simulink model "nn_12B_with_contracts"  (R2019b)
settings: Solver=FixedStepDiscrete  StartTime=0  StopTime=100  FixedStep=1  RelTol=1e-3  EnableMultiTasking=on
model workspace (MAT data in the model file):
  ContractValidatorBlocksMap = containers.Map
  ContractValidatorBlocksMap.serialization.keys = {'nn_12B_with_contracts/nn_12B_NNSpec/validator'}
  ContractValidatorBlocksMap.serialization.values{1}.block = 'nn_12B_with_contracts/nn_12B_NNSpec/validator'
  ContractValidatorBlocksMap.serialization.values{1}.assumePorts = 0
  ContractValidatorBlocksMap.serialization.values{1}.guaranteePorts = 5
  ContractValidatorBlocksMap.serialization.values{1}.modeBlocksPorts = 0
  ContractValidatorBlocksMap.serialization.values{1}.portHandles.Inport = [1930.00012207 1931.00012207 1932.00012207 1933.00012207 1934.00012207]
  ContractValidatorBlocksMap.serialization.values{1}.portHandles.Outport = 1935.00012207
  ContractValidatorBlocksMap.serialization.values{1}.portHandles.Enable = []
  ContractValidatorBlocksMap.serialization.values{1}.portHandles.Trigger = []
  ContractValidatorBlocksMap.serialization.values{1}.portHandles.State = []
  ContractValidatorBlocksMap.serialization.values{1}.portHandles.LConn = []
  ContractValidatorBlocksMap.serialization.values{1}.portHandles.RConn = []
  ContractValidatorBlocksMap.serialization.values{1}.portHandles.Ifaction = []
  ContractValidatorBlocksMap.serialization.values{1}.portHandles.Reset = []
  ContractValidatorBlocksMap.serialization.values{1}.portConnectivity(1).Type = '1'
  ContractValidatorBlocksMap.serialization.values{1}.portConnectivity(1).Position = [2170 860]
  ContractValidatorBlocksMap.serialization.values{1}.portConnectivity(1).SrcBlock = 233.00012207
  ContractValidatorBlocksMap.serialization.values{1}.portConnectivity(1).SrcPort = 0
  ContractValidatorBlocksMap.serialization.values{1}.portConnectivity(1).DstBlock = []
  ContractValidatorBlocksMap.serialization.values{1}.portConnectivity(1).DstPort = []
  ContractValidatorBlocksMap.serialization.values{1}.portConnectivity(2).Type = '2'
  ContractValidatorBlocksMap.serialization.values{1}.portConnectivity(2).Position = [2170 905]
  ContractValidatorBlocksMap.serialization.values{1}.portConnectivity(2).SrcBlock = 237.00012207
  ContractValidatorBlocksMap.serialization.values{1}.portConnectivity(2).SrcPort = 0
  ContractValidatorBlocksMap.serialization.values{1}.portConnectivity(2).DstBlock = []
  ContractValidatorBlocksMap.serialization.values{1}.portConnectivity(2).DstPort = []
  ContractValidatorBlocksMap.serialization.values{1}.portConnectivity(3).Type = '3'
  ContractValidatorBlocksMap.serialization.values{1}.portConnectivity(3).Position = [2170 950]
  ContractValidatorBlocksMap.serialization.values{1}.portConnectivity(3).SrcBlock = 241.00012207
  ContractValidatorBlocksMap.serialization.values{1}.portConnectivity(3).SrcPort = 0
  ContractValidatorBlocksMap.serialization.values{1}.portConnectivity(3).DstBlock = []
  ContractValidatorBlocksMap.serialization.values{1}.portConnectivity(3).DstPort = []
  ContractValidatorBlocksMap.serialization.values{1}.portConnectivity(4).Type = '4'
  ContractValidatorBlocksMap.serialization.values{1}.portConnectivity(4).Position = [2170 995]
  ContractValidatorBlocksMap.serialization.values{1}.portConnectivity(4).SrcBlock = 245.00012207
  ContractValidatorBlocksMap.serialization.values{1}.portConnectivity(4).SrcPort = 0
  ContractValidatorBlocksMap.serialization.values{1}.portConnectivity(4).DstBlock = []
  ContractValidatorBlocksMap.serialization.values{1}.portConnectivity(4).DstPort = []
  ContractValidatorBlocksMap.serialization.values{1}.portConnectivity(5).Type = '5'
  ContractValidatorBlocksMap.serialization.values{1}.portConnectivity(5).Position = [2170 1040]
  ContractValidatorBlocksMap.serialization.values{1}.portConnectivity(5).SrcBlock = 249.00012207
  ContractValidatorBlocksMap.serialization.values{1}.portConnectivity(5).SrcPort = 0
  ContractValidatorBlocksMap.serialization.values{1}.portConnectivity(5).DstBlock = []
  ContractValidatorBlocksMap.serialization.values{1}.portConnectivity(5).DstPort = []
  ContractValidatorBlocksMap.serialization.values{1}.portConnectivity(6).Type = '1'
  ContractValidatorBlocksMap.serialization.values{1}.portConnectivity(6).Position = [2210 950]
  ContractValidatorBlocksMap.serialization.values{1}.portConnectivity(6).SrcBlock = []
  ContractValidatorBlocksMap.serialization.values{1}.portConnectivity(6).SrcPort = []
  ContractValidatorBlocksMap.serialization.values{1}.portConnectivity(6).DstBlock = 291.00012207
  ContractValidatorBlocksMap.serialization.values{1}.portConnectivity(6).DstPort = 0
  ContractValidatorBlocksMap.serialization.uniformity = 0
  ContractValidatorBlocksMap.serialization.keyType = 'char'
  ContractValidatorBlocksMap.serialization.valueType = 'any'
undefined symbols (not defined in the file): b1, b2, b3, contractAfterSimulation, contractBeforeSimulation, ContractBlock, ContractGuaranteeBlock, ContractValidatorBlock, meaninp, meanout, oostdinp, saveValidatorParameters, stdevout, w1, w2, w3, xinmax, xinmin
libraries: cocosimLibs x4
(part 1 of 2)
settings Model: Creator=niestma  LastModifiedBy=hbourbou
settings DataIOCC: LimitDataPoints=on  SaveFormat=Array  ReturnWorkspaceOutputs=off
settings OptimizationCC: ExpressionDepthLimit=2147483647  LifeSpan=1  EfficientTunableParamExpr=on
settings DebuggingCC: UnderspecifiedInitializationDetection=Classic  MergeDetectMultiDrivingBlocksExec=none  StateNameClashWarn=warning  SFUnexpectedBacktrackingDiag=warning  SFNoUnconditionalDefaultTransitionDiag=warning  SFExecutionAtInitializationDiag=none  ArithmeticOperatorsInVariantConditions=warning
settings HardwareCC: ProdBitPerPointer=32  ProdBitPerSizeT=32  ProdBitPerPtrDiffT=32  ProdLargestAtomicFloat=None  ProdIntDivRoundTo=Undefined  ProdEndianess=Unspecified  ProdWordSize=32  ProdHWDeviceType=32-bit Generic
settings ModelReferenceCC: PropagateSignalLabelsOutOfModel=off
settings SFSimCC: SimUseLocalCustomCode=off  MATLABDynamicMemAlloc=off  CustomCodeUndefinedFunction=UseInterfaceOnly
settings RTWCC: SystemTargetFile=ert.tlc  TemplateMakefile=ert_default_tmf  GenerateReport=on  RTWUseLocalCustomCode=off  IncludeHyperlinkInReport=on  LaunchReport=on
settings CodeAppCC: IgnoreCustomStorageClasses=off  CustomSymbolStrType=$N$R$M  StateflowObjectComments=on  InternalIdentifier=Classic
settings ERTTargetCC: MultiwordLength=2048  GenerateSampleERTMain=on  ERTCustomFileTemplate=example_file_process.tlc  ConvertIfToSwitch=off  SuppressUnreachableDefaultCases=off
settings ConfigComp: CovMetricSettings=dw  CovHtmlReporting=on  CovSaveCumulativeToWorkspaceVar=on  CovSaveSingleToWorkspaceVar=on  CovExternalEMLEnable=off

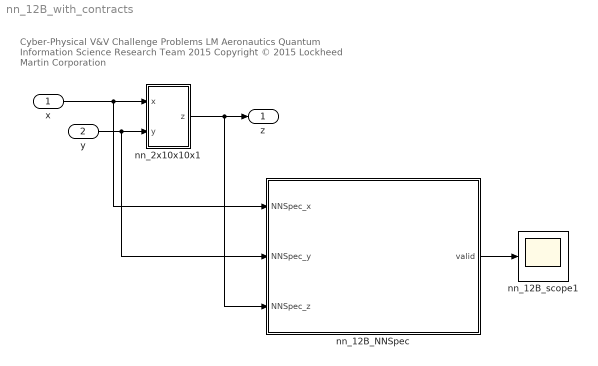
== system nn_12B_with_contracts ==
  note: Cyber-Physical V&V Challenge Problems
      | LM Aeronautics Quantum Information Science Research Team 2015
      | Copyright © 2015 Lockheed Martin Corporation
  x : Inport  OutDataTypeStr=double
  y : Inport  Port=2  OutDataTypeStr=double
  nn_12B_NNSpec : Subsystem  mask(ContractBlock){ContractBlockType=ContractBlock}
      mask init:
      | set_param(gcb, 'LinkStatus', 'none');
      mask DialogControl DescTextVar Prompt: Contract block
      mask Display:
      | text(0.5, 0.5, '{\bf\fontsize{20}Contract}', 'hor', 'center', 'texmode','on');
      | blocks = find_system(gcb, 'LookUnderMasks','all', 'SearchDepth',1,'BlockType','Inport');
      | for i = 1 : length(blocks)
      |     blockName = get_param(blocks(i), 'Name');
      |     [path, blockName] = fileparts(char(blockName));
      |     port_label('input', i, blockName);
      | end
      | 
      | blocks = find_system(gcb, 'LookUnderMasks','all', 'SearchDepth',1,'BlockType','Outport');
      | for i = 1 : length(blocks)
      |     blockName = get_param(blocks(i), 'Name');
      |     [path, blockName] = fileparts(char(blockName));
      |     port_label('output', i, blockName);
      | end
  nn_12B_scope1 : Scope
  nn_2x10x10x1 : Subsystem
  z : Outport  VectorParamsAs1DForOutWhenUnconnected=off
  wires:
  nn_2x10x10x1/1(z) -> nn_12B_NNSpec/3(NNSpec_z), z/1
  x/1 -> nn_12B_NNSpec/1(NNSpec_x), nn_2x10x10x1/1(x)
  y/1 -> nn_12B_NNSpec/2(NNSpec_y), nn_2x10x10x1/2(y)
  nn_12B_NNSpec/1(valid) -> nn_12B_scope1/1

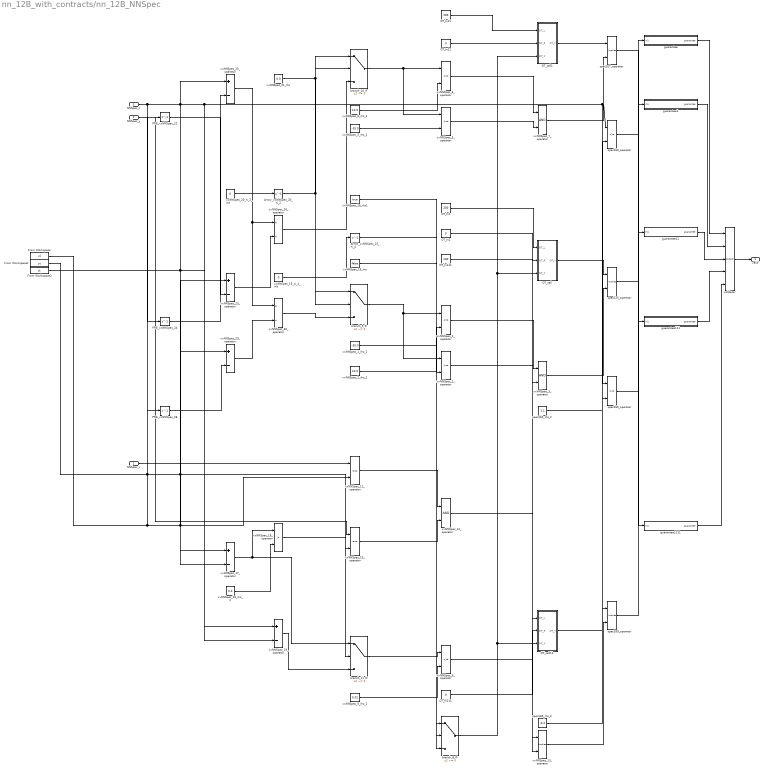
== system nn_12B_with_contracts/nn_12B_NNSpec ==
  NNSpec_x : Inport  OutDataTypeStr=double
  NNSpec_y : Inport  Port=2  OutDataTypeStr=double
  NNSpec_z : Inport  Port=3  OutDataTypeStr=double
  Arrow_xxNNSpec_15_ni_4 : Delay  DelayLength=1  InitialCondition=1
  Arrow_xxNNSpec_20_ni_2 : Delay  DelayLength=1  InitialCondition=1
  From Workspace : FromWorkspace  VariableName=xt  SampleTime=1  Interpolate=off  OutputAfterFinalValue=Holding final value
  From Workspace1 : FromWorkspace  VariableName=yt  SampleTime=1  Interpolate=off  OutputAfterFinalValue=Holding final value
  From Workspace2 : FromWorkspace  VariableName=zt  SampleTime=1  Interpolate=off  OutputAfterFinalValue=Holding final value
  OT_In1 : Constant  Value=200  OutDataTypeStr=int32
  OT_In11 : Constant  Value=200  OutDataTypeStr=int32
  OT_In111 : Constant  Value=200  OutDataTypeStr=int32
  OT_In2 : Constant  Value=0  OutDataTypeStr=int32
  OT_In21 : Constant  Value=0  OutDataTypeStr=int32
  OT_In211 : Constant  Value=0  OutDataTypeStr=int32
  OT_call : Subsystem
  OT_call1 : Subsystem
  OT_call11 : Subsystem
  PRE_xxNNSpec_22 : Delay  DelayLength=1  InitialCondition=0
  PRE_xxNNSpec_24 : Delay  DelayLength=1  InitialCondition=0
  PRE_xxNNSpec_28 : Delay  DelayLength=1  InitialCondition=0
  branch_10_IF : Switch  Criteria=u2 ~= 0
  branch_11_IF : Switch  Criteria=u2 ~= 0
  branch_8_IF : Switch  Criteria=u2 ~= 0
  branch_9_IF : Switch  Criteria=u2 ~= 0
  guarantee : Subsystem  mask(ContractGuaranteeBlock){ContractBlockType=ContractGuaranteeBlock}
      mask init:
      | set_param(gcb, 'LinkStatus', 'none');
      mask DialogControl DescTextVar Prompt: Guarantee block
  guarantee1 : Subsystem  mask(ContractGuaranteeBlock){ContractBlockType=ContractGuaranteeBlock}
      mask init:
      | set_param(gcb, 'LinkStatus', 'none');
      mask DialogControl DescTextVar Prompt: Guarantee block
  guarantee11 : Subsystem  mask(ContractGuaranteeBlock){ContractBlockType=ContractGuaranteeBlock}
      mask init:
      | set_param(gcb, 'LinkStatus', 'none');
      mask DialogControl DescTextVar Prompt: Guarantee block
  guarantee111 : Subsystem  mask(ContractGuaranteeBlock){ContractBlockType=ContractGuaranteeBlock}
      mask init:
      | set_param(gcb, 'LinkStatus', 'none');
      mask DialogControl DescTextVar Prompt: Guarantee block
  guarantee1111 : Subsystem  mask(ContractGuaranteeBlock){ContractBlockType=ContractGuaranteeBlock}
      mask init:
      | set_param(gcb, 'LinkStatus', 'none');
      mask DialogControl DescTextVar Prompt: Guarantee block
  spec160_operator : RelationalOperator  Operator=<=  OutDataTypeStr=boolean  RndMeth=Simplest
  spec160_rhs_2 : Constant  Value=1.1  OutDataTypeStr=double
  spec165_operator : RelationalOperator  OutDataTypeStr=boolean  RndMeth=Simplest
  spec165_rhs_2 : Constant  Value=-0.2  OutDataTypeStr=double
  spec189_operator : cocosimLibs/Implies  SystemSampleTime=-1  Latency=0  AutoFrameSizeCalculation=off
  spec207_operator : cocosimLibs/Implies  SystemSampleTime=-1  Latency=0  AutoFrameSizeCalculation=off
  spec225_operator : cocosimLibs/Implies  SystemSampleTime=-1  Latency=0  AutoFrameSizeCalculation=off
  validator : M-S-Function  LoadFcn=saveValidatorParameters(gcb);  InitFcn=contractBeforeSimulation();  StopFcn=contractAfterSimulation();  FunctionName=contract  mask(ContractValidatorBlock){assumePorts=0, guaranteePorts=5, modePorts=0, ContractBlockType=ContractValidatorBlock, createInportsCheckbox=off}
      mask prompts: assumePorts "Assume ports     :"; guaranteePorts "Guarantee ports :"; modePorts "Mode ports        :"; createInportsCheckbox "Create inports and connect them automatically"
      mask init:
      | set_param(gcb,'LinkStatus','none');
      | contract_callback('inputs_callback',gcb);
      mask DialogControl DescTextVar Prompt: The validator block implements the following logic: <br> <br> <b>Sofar</b>(assume<sub>1</sub> <b>&#8743;</b> assume<sub>2</sub> <b>&#8743;</b> ... assume<sub>k</sub>) <b>&rarr;</b> (guarantee<sub>1</sub> <b>&#8743;</b> guarantee<sub>2</sub> <b>&#8743;</b> ... guarantee<sub>m</sub> <b>&#8743;</b>  mode<sub>1</sub> <b>&#8743;</b> mode<sub>2</sub> <b>&#8743;</b> ... <b>&#8743;</b> mode<sub>n</sub> )<br> where mode<sub>i</sub> = require<sub>i</sub> <b>&rarr;</b> ensure<sub>i</sub>
      mask Display:
      | color('black');
      | port_label('input',1,'guarantee');
      | port_label('input',2,'guarantee');
      | port_label('input',3,'guarantee');
      | port_label('input',4,'guarantee');
      | port_label('input',5,'guarantee');
      | port_label('output',1,'valid');
  xxNNSpec_10_operator : RelationalOperator  Operator===  OutDataTypeStr=boolean  RndMeth=Simplest
  xxNNSpec_11_operator : RelationalOperator  Operator===  OutDataTypeStr=boolean  RndMeth=Simplest
  xxNNSpec_12_operator : Logic  AllPortsSameDT=off  OutDataTypeStr=boolean
  xxNNSpec_13_operator : cocosimLibs/Implies  SystemSampleTime=-1  Latency=0  AutoFrameSizeCalculation=off
  xxNNSpec_15_ni_4_init : Constant  Value=0  OutDataTypeStr=boolean
  xxNNSpec_16_rhs : Constant  Value=false  OutDataTypeStr=boolean
  xxNNSpec_16_rhs1 : Constant  Value=true  OutDataTypeStr=boolean
  xxNNSpec_17_operator : Sum  Inputs=+-  OutDataTypeStr=double
  xxNNSpec_18_operator : RelationalOperator  Operator=>  OutDataTypeStr=boolean  RndMeth=Simplest
  xxNNSpec_18_rhs_2 : Constant  Value=0.0  OutDataTypeStr=double
  xxNNSpec_19_operator : Sum  Inputs=+-  OutDataTypeStr=double
  xxNNSpec_1_operator : RelationalOperator  OutDataTypeStr=boolean  RndMeth=Simplest
  xxNNSpec_1_rhs_2 : Constant  Value=-35.0  OutDataTypeStr=double
  xxNNSpec_20_ni_2_init : Constant  Value=0  OutDataTypeStr=boolean
  xxNNSpec_21_rhs : Constant  Value=0.0  OutDataTypeStr=double
  xxNNSpec_23_operator : Sum  Inputs=+-  OutDataTypeStr=double
  xxNNSpec_25_operator : Sum  Inputs=+-  OutDataTypeStr=double
  xxNNSpec_26_operator : Product  Inputs=*/  OutDataTypeStr=double
  xxNNSpec_29_operator : Sum  Inputs=+-  OutDataTypeStr=double
  xxNNSpec_2_operator : RelationalOperator  Operator=<=  OutDataTypeStr=boolean  RndMeth=Simplest
  xxNNSpec_2_rhs_2 : Constant  Value=10.0  OutDataTypeStr=double
  xxNNSpec_30_operator : Product  Inputs=*/  OutDataTypeStr=double
  xxNNSpec_3_operator : Logic  AllPortsSameDT=off  OutDataTypeStr=boolean
  xxNNSpec_5_operator : RelationalOperator  OutDataTypeStr=boolean  RndMeth=Simplest
  xxNNSpec_5_rhs_2 : Constant  Value=-35.0  OutDataTypeStr=double
  xxNNSpec_6_operator : RelationalOperator  Operator=<=  OutDataTypeStr=boolean  RndMeth=Simplest
  xxNNSpec_6_rhs_2 : Constant  Value=10.0  OutDataTypeStr=double
  xxNNSpec_7_operator : Logic  AllPortsSameDT=off  OutDataTypeStr=boolean
  xxNNSpec_9_operator : RelationalOperator  Operator=<=  OutDataTypeStr=boolean  RndMeth=Simplest
  xxNNSpec_9_rhs_2 : Constant  Value=0.01  OutDataTypeStr=double
  valid : Outport
  wires:
  validator/1 -> valid/1
  xxNNSpec_9_rhs_2/1 -> xxNNSpec_9_operator/2
  branch_11_IF/1 -> xxNNSpec_9_operator/1
  xxNNSpec_5_operator/1 -> xxNNSpec_7_operator/2
  xxNNSpec_6_operator/1 -> xxNNSpec_7_operator/1
  xxNNSpec_6_rhs_2/1 -> xxNNSpec_6_operator/2
  xxNNSpec_5_rhs_2/1 -> xxNNSpec_5_operator/2
  xxNNSpec_1_operator/1 -> xxNNSpec_3_operator/2
  xxNNSpec_2_operator/1 -> xxNNSpec_3_operator/1
  xxNNSpec_29_operator/1 -> xxNNSpec_30_operator/2
  xxNNSpec_2_rhs_2/1 -> xxNNSpec_2_operator/2
  PRE_xxNNSpec_28/1 -> xxNNSpec_29_operator/2
  xxNNSpec_23_operator/1 -> xxNNSpec_26_operator/2
  PRE_xxNNSpec_24/1 -> xxNNSpec_25_operator/2
  PRE_xxNNSpec_22/1 -> xxNNSpec_23_operator/2
  xxNNSpec_1_rhs_2/1 -> xxNNSpec_1_operator/2
  xxNNSpec_18_rhs_2/1 -> xxNNSpec_18_operator/2
  xxNNSpec_9_operator/1 -> xxNNSpec_13_operator/2
  xxNNSpec_12_operator/1 -> xxNNSpec_13_operator/1
  xxNNSpec_10_operator/1 -> xxNNSpec_12_operator/2
  xxNNSpec_11_operator/1 -> xxNNSpec_12_operator/1
  NNSpec_x/1 -> xxNNSpec_11_operator/1
  NNSpec_y/1 -> xxNNSpec_10_operator/1
  guarantee1111/1(guarantee) -> validator/5
  guarantee111/1(guarantee) -> validator/4
  guarantee11/1(guarantee) -> validator/3
  guarantee1/1(guarantee) -> validator/2
  guarantee/1(guarantee) -> validator/1
  xxNNSpec_3_operator/1 -> spec225_operator/2
  OT_call/1(OT_Y) -> spec225_operator/1
  xxNNSpec_7_operator/1 -> spec207_operator/2
  OT_call1/1(OT_Y) -> spec207_operator/1
  xxNNSpec_13_operator/1 -> spec189_operator/2
  OT_call11/1(OT_Y) -> spec189_operator/1
  spec165_rhs_2/1 -> spec165_operator/2
  spec160_rhs_2/1 -> spec160_operator/2
  spec225_operator/1 -> guarantee1111/1(In1)
  spec207_operator/1 -> guarantee111/1(In1)
  spec189_operator/1 -> guarantee11/1(In1)
  spec165_operator/1 -> guarantee1/1(In1)
  spec160_operator/1 -> guarantee/1(In1)
  xxNNSpec_30_operator/1 -> branch_9_IF/3
  xxNNSpec_16_rhs/1 -> branch_8_IF/3
  Arrow_xxNNSpec_15_ni_4/1 -> branch_8_IF/2
  xxNNSpec_16_rhs1/1 -> branch_8_IF/1
  xxNNSpec_19_operator/1 -> branch_11_IF/3
  xxNNSpec_18_operator/1 -> branch_11_IF/2
  xxNNSpec_26_operator/1 -> branch_10_IF/3
  OT_In211/1 -> OT_call11/2(OT_R)
  OT_In111/1 -> OT_call11/1(OT_L)
  OT_In21/1 -> OT_call1/2(OT_R)
  OT_In11/1 -> OT_call1/1(OT_L)
  OT_In2/1 -> OT_call/2(OT_R)
  OT_In1/1 -> OT_call/1(OT_L)
  xxNNSpec_20_ni_2_init/1 -> Arrow_xxNNSpec_20_ni_2/1
  xxNNSpec_15_ni_4_init/1 -> Arrow_xxNNSpec_15_ni_4/1
  NNSpec_z/1 -> spec165_operator/1, spec160_operator/1, xxNNSpec_19_operator/1, xxNNSpec_25_operator/1, xxNNSpec_17_operator/2, PRE_xxNNSpec_24/1
  From Workspace1/1 -> xxNNSpec_23_operator/1, xxNNSpec_10_operator/2, PRE_xxNNSpec_22/1
  From Workspace/1 -> xxNNSpec_29_operator/1, xxNNSpec_11_operator/2, PRE_xxNNSpec_28/1
  xxNNSpec_17_operator/1 -> xxNNSpec_18_operator/1, branch_11_IF/1
  From Workspace2/1 -> xxNNSpec_19_operator/2, xxNNSpec_17_operator/1
  branch_10_IF/1 -> xxNNSpec_6_operator/1, xxNNSpec_5_operator/1
  xxNNSpec_21_rhs/1 -> branch_9_IF/1, branch_10_IF/1
  Arrow_xxNNSpec_20_ni_2/1 -> branch_9_IF/2, branch_10_IF/2
  xxNNSpec_25_operator/1 -> xxNNSpec_30_operator/1, xxNNSpec_26_operator/1
  branch_9_IF/1 -> xxNNSpec_2_operator/1, xxNNSpec_1_operator/1
  branch_8_IF/1 -> OT_call1/3(OT_X), OT_call/3(OT_X), OT_call11/3(OT_X)

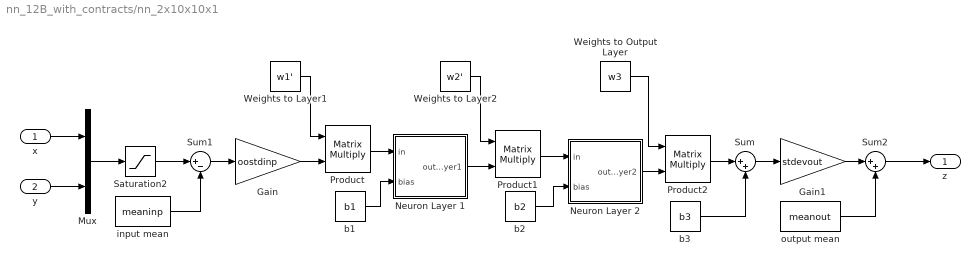
== system nn_12B_with_contracts/nn_2x10x10x1 ==
  x : Inport
  y : Inport  Port=2
  Gain : Gain  Gain=oostdinp
  Gain1 : Gain  Gain=stdevout
  Mux : Mux  Inputs=2
  Neuron Layer 1 : Subsystem
  Neuron Layer 2 : Subsystem
  Product : Product  Multiplication=Matrix(*)  RndMeth=Zero
  Product1 : Product  Multiplication=Matrix(*)  RndMeth=Zero
  Product2 : Product  Multiplication=Matrix(*)  RndMeth=Zero
  Saturation2 : Saturate  UpperLimit=xinmax  LowerLimit=xinmin
  Sum : Sum  Inputs=|++
  Sum1 : Sum  Inputs=|+-
  Sum2 : Sum  Inputs=|++
  Weights to Layer1 : Constant  Value=w1'  VectorParams1D=off
  Weights to Layer2 : Constant  Value=w2'  VectorParams1D=off
  Weights to Output Layer : Constant  Value=w3  VectorParams1D=off
  b1 : Constant  Value=b1
  b2 : Constant  Value=b2
  b3 : Constant  Value=b3
  input mean : Constant  Value=meaninp
  output mean : Constant  Value=meanout
  z : Outport  VectorParamsAs1DForOutWhenUnconnected=off
  wires:
  Product1/1 -> Neuron Layer 2/1(in)
  b2/1 -> Neuron Layer 2/2(bias)
  x/1 -> Mux/1
  b1/1 -> Neuron Layer 1/2(bias)
  b3/1 -> Sum/2
  y/1 -> Mux/2
  Weights to Layer1/1 -> Product/1
  Weights to Layer2/1 -> Product1/1
  Product/1 -> Neuron Layer 1/1(in)
  Neuron Layer 1/1(output layer1) -> Product1/2
  Weights to Output Layer/1 -> Product2/1
  Neuron Layer 2/1(output layer2) -> Product2/2
  Product2/1 -> Sum/1
  Mux/1 -> Saturation2/1
  Saturation2/1 -> Sum1/1
  input mean/1 -> Sum1/2
  Gain/1 -> Product/2
  Sum1/1 -> Gain/1
  Sum/1 -> Gain1/1
  Gain1/1 -> Sum2/1
  Sum2/1 -> z/1
  output mean/1 -> Sum2/2

== system nn_12B_with_contracts/nn_12B_NNSpec/OT_call ==
  OT_L : Inport
  OT_R : Inport  Port=2
  OT_X : Inport  Port=3  OutDataTypeStr=boolean
  OTlore_call : Subsystem
  delay_call : Subsystem
  xxOT_1_operator : Sum  Inputs=+-  OutDataTypeStr=int32
  OT_Y : Outport
  wires:
  OTlore_call/1(OTlore_Y) -> OT_Y/1
  OT_L/1 -> xxOT_1_operator/1
  OT_X/1 -> delay_call/1(delay_X)
  delay_call/1(delay_Y) -> OTlore_call/2(OTlore_X)
  xxOT_1_operator/1 -> OTlore_call/1(OTlore_N)
  OT_R/1 -> xxOT_1_operator/2, delay_call/2(delay_R)

== system nn_12B_with_contracts/nn_12B_NNSpec/OT_call1 ==
  OT_L : Inport
  OT_R : Inport  Port=2
  OT_X : Inport  Port=3  OutDataTypeStr=boolean
  OTlore_call : Subsystem
  delay_call : Subsystem
  xxOT_1_operator : Sum  Inputs=+-  OutDataTypeStr=int32
  OT_Y : Outport
  wires:
  OTlore_call/1(OTlore_Y) -> OT_Y/1
  OT_L/1 -> xxOT_1_operator/1
  OT_X/1 -> delay_call/1(delay_X)
  delay_call/1(delay_Y) -> OTlore_call/2(OTlore_X)
  xxOT_1_operator/1 -> OTlore_call/1(OTlore_N)
  OT_R/1 -> xxOT_1_operator/2, delay_call/2(delay_R)

== system nn_12B_with_contracts/nn_12B_NNSpec/OT_call11 ==
  OT_L : Inport
  OT_R : Inport  Port=2
  OT_X : Inport  Port=3  OutDataTypeStr=boolean
  OTlore_call : Subsystem
  delay_call : Subsystem
  xxOT_1_operator : Sum  Inputs=+-  OutDataTypeStr=int32
  OT_Y : Outport
  wires:
  OTlore_call/1(OTlore_Y) -> OT_Y/1
  OT_L/1 -> xxOT_1_operator/1
  OT_X/1 -> delay_call/1(delay_X)
  delay_call/1(delay_Y) -> OTlore_call/2(OTlore_X)
  xxOT_1_operator/1 -> OTlore_call/1(OTlore_N)
  OT_R/1 -> xxOT_1_operator/2, delay_call/2(delay_R)

== system nn_12B_with_contracts/nn_12B_NNSpec/guarantee ==
  In1 : Inport
  guarantee : Outport  OutDataTypeStr=boolean
  wires:
  In1/1 -> guarantee/1

== system nn_12B_with_contracts/nn_12B_NNSpec/guarantee1 ==
  In1 : Inport
  guarantee : Outport  OutDataTypeStr=boolean
  wires:
  In1/1 -> guarantee/1

== system nn_12B_with_contracts/nn_12B_NNSpec/guarantee11 ==
  In1 : Inport
  guarantee : Outport  OutDataTypeStr=boolean
  wires:
  In1/1 -> guarantee/1

== system nn_12B_with_contracts/nn_12B_NNSpec/guarantee111 ==
  In1 : Inport
  guarantee : Outport  OutDataTypeStr=boolean
  wires:
  In1/1 -> guarantee/1

== system nn_12B_with_contracts/nn_12B_NNSpec/guarantee1111 ==
  In1 : Inport
  guarantee : Outport  OutDataTypeStr=boolean
  wires:
  In1/1 -> guarantee/1

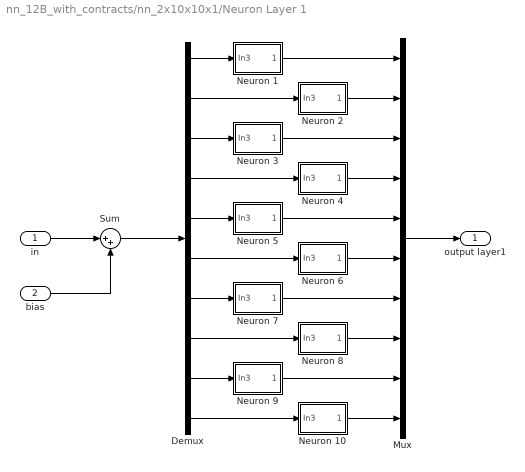
== system nn_12B_with_contracts/nn_2x10x10x1/Neuron Layer 1 ==
  in : Inport
  bias : Inport  Port=2
  Demux : Demux  Outputs=10
  Mux : Mux  Inputs=10
  Neuron 1 : Subsystem
  Neuron 10 : Subsystem
  Neuron 2 : Subsystem
  Neuron 3 : Subsystem
  Neuron 4 : Subsystem
  Neuron 5 : Subsystem
  Neuron 6 : Subsystem
  Neuron 7 : Subsystem
  Neuron 8 : Subsystem
  Neuron 9 : Subsystem
  Sum : Sum  Inputs=|++
  output layer1 : Outport  VectorParamsAs1DForOutWhenUnconnected=off
  wires:
  bias/1 -> Sum/2
  in/1 -> Sum/1
  Sum/1 -> Demux/1
  Demux/1 -> Neuron 1/1(In3)
  Neuron 1/1(Out1) -> Mux/1
  Mux/1 -> output layer1/1
  Neuron 2/1(Out1) -> Mux/2
  Demux/2 -> Neuron 2/1(In3)
  Demux/3 -> Neuron 3/1(In3)
  Neuron 3/1(Out1) -> Mux/3
  Demux/4 -> Neuron 4/1(In3)
  Neuron 4/1(Out1) -> Mux/4
  Demux/5 -> Neuron 5/1(In3)
  Neuron 5/1(Out1) -> Mux/5
  Demux/6 -> Neuron 6/1(In3)
  Demux/7 -> Neuron 7/1(In3)
  Neuron 7/1(Out1) -> Mux/7
  Demux/8 -> Neuron 8/1(In3)
  Neuron 6/1(Out1) -> Mux/6
  Neuron 8/1(Out1) -> Mux/8
  Demux/9 -> Neuron 9/1(In3)
  Neuron 9/1(Out1) -> Mux/9
  Demux/10 -> Neuron 10/1(In3)
  Neuron 10/1(Out1) -> Mux/10

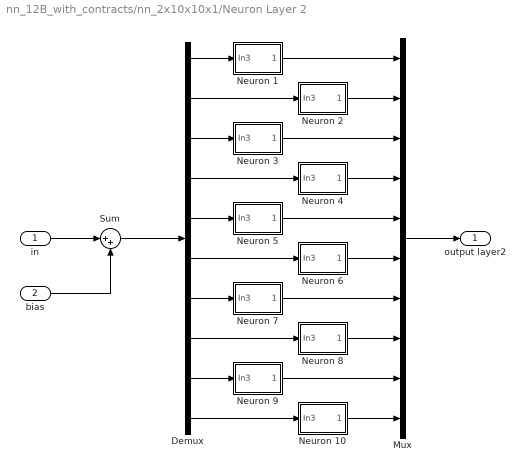
== system nn_12B_with_contracts/nn_2x10x10x1/Neuron Layer 2 ==
  in : Inport
  bias : Inport  Port=2
  Demux : Demux  Outputs=10
  Mux : Mux  Inputs=10
  Neuron 1 : Subsystem
  Neuron 10 : Subsystem
  Neuron 2 : Subsystem
  Neuron 3 : Subsystem
  Neuron 4 : Subsystem
  Neuron 5 : Subsystem
  Neuron 6 : Subsystem
  Neuron 7 : Subsystem
  Neuron 8 : Subsystem
  Neuron 9 : Subsystem
  Sum : Sum  Inputs=|++
  output layer2 : Outport  VectorParamsAs1DForOutWhenUnconnected=off
  wires:
  bias/1 -> Sum/2
  in/1 -> Sum/1
  Sum/1 -> Demux/1
  Demux/1 -> Neuron 1/1(In3)
  Neuron 1/1(Out1) -> Mux/1
  Mux/1 -> output layer2/1
  Neuron 2/1(Out1) -> Mux/2
  Demux/2 -> Neuron 2/1(In3)
  Demux/3 -> Neuron 3/1(In3)
  Neuron 3/1(Out1) -> Mux/3
  Demux/4 -> Neuron 4/1(In3)
  Neuron 4/1(Out1) -> Mux/4
  Demux/5 -> Neuron 5/1(In3)
  Neuron 5/1(Out1) -> Mux/5
  Demux/6 -> Neuron 6/1(In3)
  Demux/7 -> Neuron 7/1(In3)
  Neuron 7/1(Out1) -> Mux/7
  Demux/8 -> Neuron 8/1(In3)
  Neuron 6/1(Out1) -> Mux/6
  Neuron 8/1(Out1) -> Mux/8
  Demux/9 -> Neuron 9/1(In3)
  Neuron 9/1(Out1) -> Mux/9
  Demux/10 -> Neuron 10/1(In3)
  Neuron 10/1(Out1) -> Mux/10

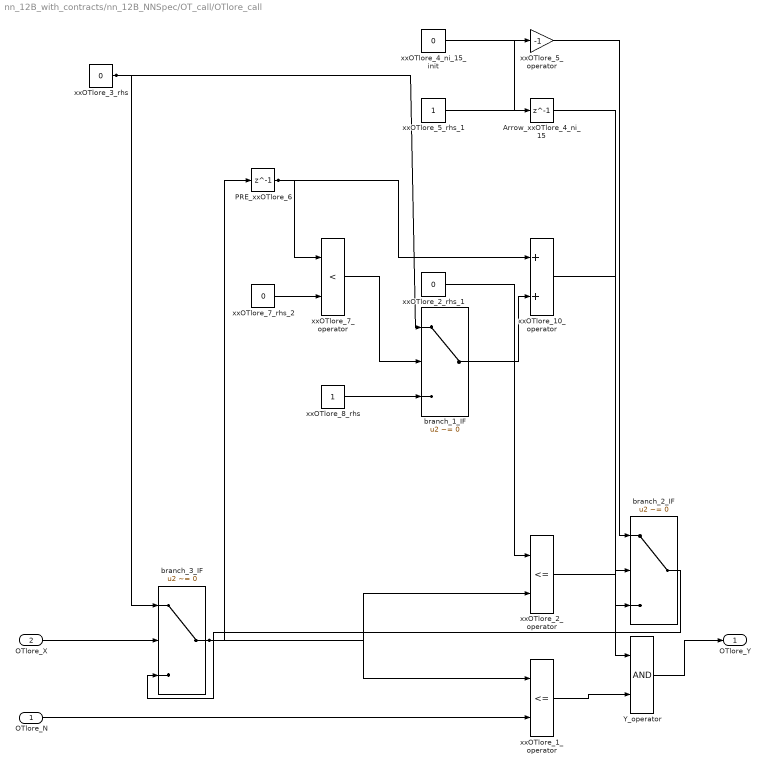
== system nn_12B_with_contracts/nn_12B_NNSpec/OT_call/OTlore_call ==
  OTlore_N : Inport
  OTlore_X : Inport  Port=2  OutDataTypeStr=boolean
  Arrow_xxOTlore_4_ni_15 : Delay  DelayLength=1  InitialCondition=1
  PRE_xxOTlore_6 : Delay  DelayLength=1  InitialCondition=0
  Y_operator : Logic  AllPortsSameDT=off  OutDataTypeStr=boolean
  branch_1_IF : Switch  Criteria=u2 ~= 0
  branch_2_IF : Switch  Criteria=u2 ~= 0
  branch_3_IF : Switch  Criteria=u2 ~= 0
  xxOTlore_10_operator : Sum  OutDataTypeStr=int32
  xxOTlore_1_operator : RelationalOperator  Operator=<=  OutDataTypeStr=boolean  RndMeth=Simplest
  xxOTlore_2_operator : RelationalOperator  Operator=<=  OutDataTypeStr=boolean  RndMeth=Simplest
  xxOTlore_2_rhs_1 : Constant  Value=0  OutDataTypeStr=int32
  xxOTlore_3_rhs : Constant  Value=0  OutDataTypeStr=Inherit: Inherit via back propagation
  xxOTlore_4_ni_15_init : Constant  Value=0  OutDataTypeStr=boolean
  xxOTlore_5_operator : Gain  Gain=-1  OutDataTypeStr=int32
  xxOTlore_5_rhs_1 : Constant  OutDataTypeStr=int32
  xxOTlore_7_operator : RelationalOperator  Operator=<  OutDataTypeStr=boolean  RndMeth=Simplest
  xxOTlore_7_rhs_2 : Constant  Value=0  OutDataTypeStr=int32
  xxOTlore_8_rhs : Constant  OutDataTypeStr=Inherit: Inherit via back propagation
  OTlore_Y : Outport
  wires:
  Y_operator/1 -> OTlore_Y/1
  xxOTlore_7_rhs_2/1 -> xxOTlore_7_operator/2
  xxOTlore_5_rhs_1/1 -> xxOTlore_5_operator/1
  xxOTlore_2_rhs_1/1 -> xxOTlore_2_operator/1
  OTlore_N/1 -> xxOTlore_1_operator/2
  branch_1_IF/1 -> xxOTlore_10_operator/2
  branch_2_IF/1 -> branch_3_IF/3
  OTlore_X/1 -> branch_3_IF/2
  xxOTlore_10_operator/1 -> branch_2_IF/3
  Arrow_xxOTlore_4_ni_15/1 -> branch_2_IF/2
  xxOTlore_5_operator/1 -> branch_2_IF/1
  xxOTlore_8_rhs/1 -> branch_1_IF/3
  xxOTlore_7_operator/1 -> branch_1_IF/2
  xxOTlore_1_operator/1 -> Y_operator/2
  xxOTlore_2_operator/1 -> Y_operator/1
  xxOTlore_4_ni_15_init/1 -> Arrow_xxOTlore_4_ni_15/1
  branch_3_IF/1 -> xxOTlore_2_operator/2, xxOTlore_1_operator/1, PRE_xxOTlore_6/1
  PRE_xxOTlore_6/1 -> xxOTlore_7_operator/1, xxOTlore_10_operator/1
  xxOTlore_3_rhs/1 -> branch_3_IF/1, branch_1_IF/1

== system nn_12B_with_contracts/nn_12B_NNSpec/OT_call/delay_call ==
  delay_X : Inport  OutDataTypeStr=boolean
  delay_R : Inport  Port=2
  delay_Y : Outport
  wires:
  delay_X/1 -> delay_Y/1
  delay_R/1 -> [delay_R]

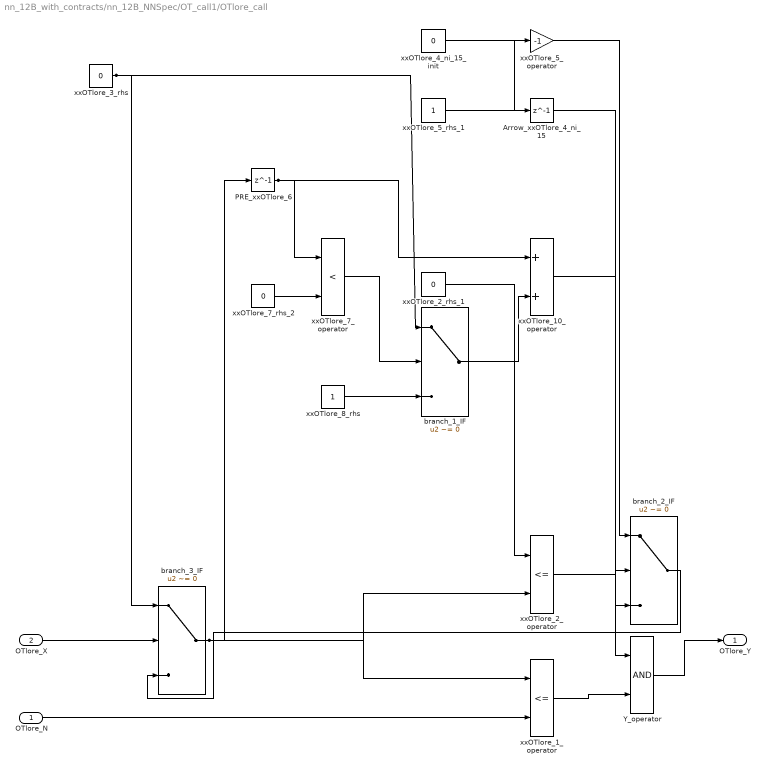
== system nn_12B_with_contracts/nn_12B_NNSpec/OT_call1/OTlore_call ==
  OTlore_N : Inport
  OTlore_X : Inport  Port=2  OutDataTypeStr=boolean
  Arrow_xxOTlore_4_ni_15 : Delay  DelayLength=1  InitialCondition=1
  PRE_xxOTlore_6 : Delay  DelayLength=1  InitialCondition=0
  Y_operator : Logic  AllPortsSameDT=off  OutDataTypeStr=boolean
  branch_1_IF : Switch  Criteria=u2 ~= 0
  branch_2_IF : Switch  Criteria=u2 ~= 0
  branch_3_IF : Switch  Criteria=u2 ~= 0
  xxOTlore_10_operator : Sum  OutDataTypeStr=int32
  xxOTlore_1_operator : RelationalOperator  Operator=<=  OutDataTypeStr=boolean  RndMeth=Simplest
  xxOTlore_2_operator : RelationalOperator  Operator=<=  OutDataTypeStr=boolean  RndMeth=Simplest
  xxOTlore_2_rhs_1 : Constant  Value=0  OutDataTypeStr=int32
  xxOTlore_3_rhs : Constant  Value=0  OutDataTypeStr=Inherit: Inherit via back propagation
  xxOTlore_4_ni_15_init : Constant  Value=0  OutDataTypeStr=boolean
  xxOTlore_5_operator : Gain  Gain=-1  OutDataTypeStr=int32
  xxOTlore_5_rhs_1 : Constant  OutDataTypeStr=int32
  xxOTlore_7_operator : RelationalOperator  Operator=<  OutDataTypeStr=boolean  RndMeth=Simplest
  xxOTlore_7_rhs_2 : Constant  Value=0  OutDataTypeStr=int32
  xxOTlore_8_rhs : Constant  OutDataTypeStr=Inherit: Inherit via back propagation
  OTlore_Y : Outport
  wires:
  Y_operator/1 -> OTlore_Y/1
  xxOTlore_7_rhs_2/1 -> xxOTlore_7_operator/2
  xxOTlore_5_rhs_1/1 -> xxOTlore_5_operator/1
  xxOTlore_2_rhs_1/1 -> xxOTlore_2_operator/1
  OTlore_N/1 -> xxOTlore_1_operator/2
  branch_1_IF/1 -> xxOTlore_10_operator/2
  branch_2_IF/1 -> branch_3_IF/3
  OTlore_X/1 -> branch_3_IF/2
  xxOTlore_10_operator/1 -> branch_2_IF/3
  Arrow_xxOTlore_4_ni_15/1 -> branch_2_IF/2
  xxOTlore_5_operator/1 -> branch_2_IF/1
  xxOTlore_8_rhs/1 -> branch_1_IF/3
  xxOTlore_7_operator/1 -> branch_1_IF/2
  xxOTlore_1_operator/1 -> Y_operator/2
  xxOTlore_2_operator/1 -> Y_operator/1
  xxOTlore_4_ni_15_init/1 -> Arrow_xxOTlore_4_ni_15/1
  branch_3_IF/1 -> xxOTlore_2_operator/2, xxOTlore_1_operator/1, PRE_xxOTlore_6/1
  PRE_xxOTlore_6/1 -> xxOTlore_7_operator/1, xxOTlore_10_operator/1
  xxOTlore_3_rhs/1 -> branch_3_IF/1, branch_1_IF/1

== system nn_12B_with_contracts/nn_12B_NNSpec/OT_call1/delay_call ==
  delay_X : Inport  OutDataTypeStr=boolean
  delay_R : Inport  Port=2
  delay_Y : Outport
  wires:
  delay_X/1 -> delay_Y/1
  delay_R/1 -> [delay_R]

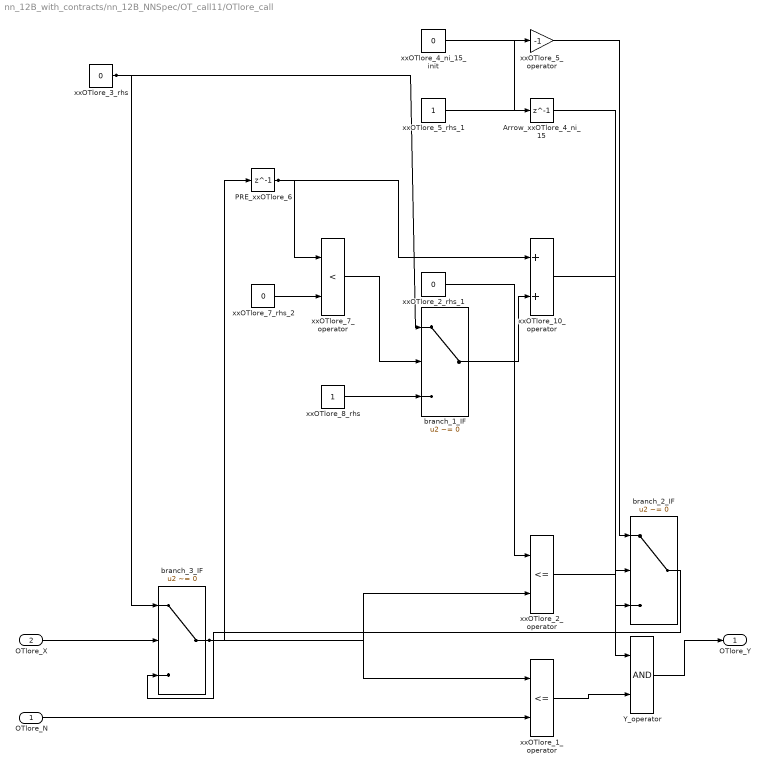
== system nn_12B_with_contracts/nn_12B_NNSpec/OT_call11/OTlore_call ==
  OTlore_N : Inport
  OTlore_X : Inport  Port=2  OutDataTypeStr=boolean
  Arrow_xxOTlore_4_ni_15 : Delay  DelayLength=1  InitialCondition=1
  PRE_xxOTlore_6 : Delay  DelayLength=1  InitialCondition=0
  Y_operator : Logic  AllPortsSameDT=off  OutDataTypeStr=boolean
  branch_1_IF : Switch  Criteria=u2 ~= 0
  branch_2_IF : Switch  Criteria=u2 ~= 0
  branch_3_IF : Switch  Criteria=u2 ~= 0
  xxOTlore_10_operator : Sum  OutDataTypeStr=int32
  xxOTlore_1_operator : RelationalOperator  Operator=<=  OutDataTypeStr=boolean  RndMeth=Simplest
  xxOTlore_2_operator : RelationalOperator  Operator=<=  OutDataTypeStr=boolean  RndMeth=Simplest
  xxOTlore_2_rhs_1 : Constant  Value=0  OutDataTypeStr=int32
  xxOTlore_3_rhs : Constant  Value=0  OutDataTypeStr=Inherit: Inherit via back propagation
  xxOTlore_4_ni_15_init : Constant  Value=0  OutDataTypeStr=boolean
  xxOTlore_5_operator : Gain  Gain=-1  OutDataTypeStr=int32
  xxOTlore_5_rhs_1 : Constant  OutDataTypeStr=int32
  xxOTlore_7_operator : RelationalOperator  Operator=<  OutDataTypeStr=boolean  RndMeth=Simplest
  xxOTlore_7_rhs_2 : Constant  Value=0  OutDataTypeStr=int32
  xxOTlore_8_rhs : Constant  OutDataTypeStr=Inherit: Inherit via back propagation
  OTlore_Y : Outport
  wires:
  Y_operator/1 -> OTlore_Y/1
  xxOTlore_7_rhs_2/1 -> xxOTlore_7_operator/2
  xxOTlore_5_rhs_1/1 -> xxOTlore_5_operator/1
  xxOTlore_2_rhs_1/1 -> xxOTlore_2_operator/1
  OTlore_N/1 -> xxOTlore_1_operator/2
  branch_1_IF/1 -> xxOTlore_10_operator/2
  branch_2_IF/1 -> branch_3_IF/3
  OTlore_X/1 -> branch_3_IF/2
  xxOTlore_10_operator/1 -> branch_2_IF/3
  Arrow_xxOTlore_4_ni_15/1 -> branch_2_IF/2
  xxOTlore_5_operator/1 -> branch_2_IF/1
  xxOTlore_8_rhs/1 -> branch_1_IF/3
  xxOTlore_7_operator/1 -> branch_1_IF/2
  xxOTlore_1_operator/1 -> Y_operator/2
  xxOTlore_2_operator/1 -> Y_operator/1
  xxOTlore_4_ni_15_init/1 -> Arrow_xxOTlore_4_ni_15/1
  branch_3_IF/1 -> xxOTlore_2_operator/2, xxOTlore_1_operator/1, PRE_xxOTlore_6/1
  PRE_xxOTlore_6/1 -> xxOTlore_7_operator/1, xxOTlore_10_operator/1
  xxOTlore_3_rhs/1 -> branch_3_IF/1, branch_1_IF/1

== system nn_12B_with_contracts/nn_12B_NNSpec/OT_call11/delay_call ==
  delay_X : Inport  OutDataTypeStr=boolean
  delay_R : Inport  Port=2
  delay_Y : Outport
  wires:
  delay_X/1 -> delay_Y/1
  delay_R/1 -> [delay_R]

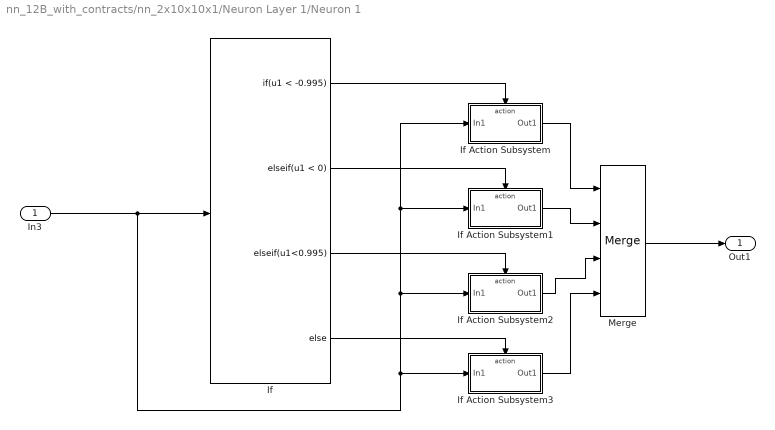
== system nn_12B_with_contracts/nn_2x10x10x1/Neuron Layer 1/Neuron 1 ==
  In3 : Inport
  If : If  IfExpression=u1 < -0.995  ElseIfExpressions=u1 < 0, u1<0.995
  If Action Subsystem : Subsystem  TreatAsAtomicUnit=on
  If Action Subsystem1 : Subsystem  TreatAsAtomicUnit=on
  If Action Subsystem2 : Subsystem  TreatAsAtomicUnit=on
  If Action Subsystem3 : Subsystem  TreatAsAtomicUnit=on
  Merge : Merge  Inputs=4
  Out1 : Outport  VectorParamsAs1DForOutWhenUnconnected=off
  wires:
  If/1 -> If Action Subsystem/Action
  If/2 -> If Action Subsystem1/Action
  If/3 -> If Action Subsystem2/Action
  If/4 -> If Action Subsystem3/Action
  If Action Subsystem/1(Out1) -> Merge/1
  If Action Subsystem3/1(Out1) -> Merge/4
  If Action Subsystem1/1(Out1) -> Merge/2
  If Action Subsystem2/1(Out1) -> Merge/3
  In3/1 -> If Action Subsystem3/1(In1), If Action Subsystem2/1(In1), If Action Subsystem1/1(In1), If Action Subsystem/1(In1), If/1
  Merge/1 -> Out1/1

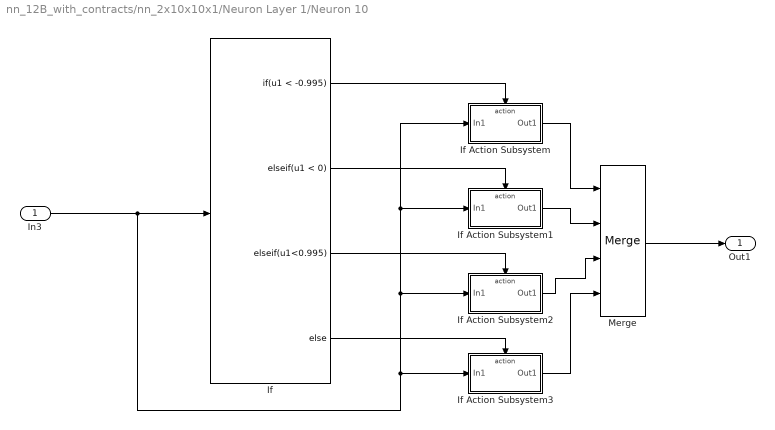
== system nn_12B_with_contracts/nn_2x10x10x1/Neuron Layer 1/Neuron 10 ==
  In3 : Inport
  If : If  IfExpression=u1 < -0.995  ElseIfExpressions=u1 < 0, u1<0.995
  If Action Subsystem : Subsystem  TreatAsAtomicUnit=on
  If Action Subsystem1 : Subsystem  TreatAsAtomicUnit=on
  If Action Subsystem2 : Subsystem  TreatAsAtomicUnit=on
  If Action Subsystem3 : Subsystem  TreatAsAtomicUnit=on
  Merge : Merge  Inputs=4
  Out1 : Outport  VectorParamsAs1DForOutWhenUnconnected=off
  wires:
  Merge/1 -> Out1/1
  In3/1 -> If/1, If Action Subsystem/1(In1), If Action Subsystem1/1(In1), If Action Subsystem2/1(In1), If Action Subsystem3/1(In1)
  If Action Subsystem2/1(Out1) -> Merge/3
  If Action Subsystem1/1(Out1) -> Merge/2
  If Action Subsystem3/1(Out1) -> Merge/4
  If Action Subsystem/1(Out1) -> Merge/1
  If/4 -> If Action Subsystem3/Action
  If/3 -> If Action Subsystem2/Action
  If/2 -> If Action Subsystem1/Action
  If/1 -> If Action Subsystem/Action

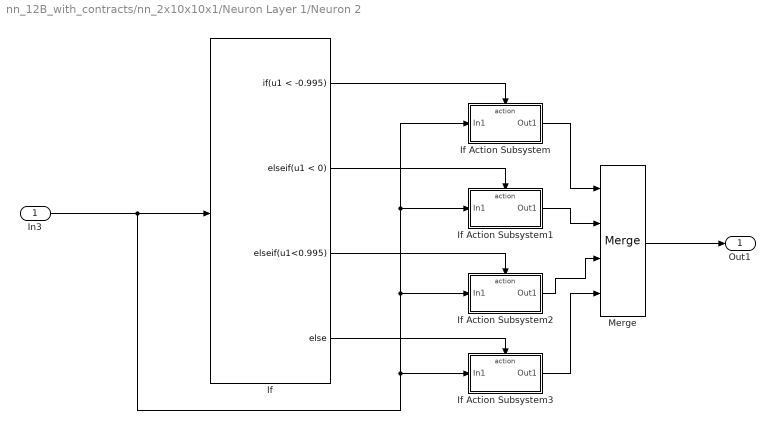
== system nn_12B_with_contracts/nn_2x10x10x1/Neuron Layer 1/Neuron 2 ==
  In3 : Inport
  If : If  IfExpression=u1 < -0.995  ElseIfExpressions=u1 < 0, u1<0.995
  If Action Subsystem : Subsystem  TreatAsAtomicUnit=on
  If Action Subsystem1 : Subsystem  TreatAsAtomicUnit=on
  If Action Subsystem2 : Subsystem  TreatAsAtomicUnit=on
  If Action Subsystem3 : Subsystem  TreatAsAtomicUnit=on
  Merge : Merge  Inputs=4
  Out1 : Outport  VectorParamsAs1DForOutWhenUnconnected=off
  wires:
  Merge/1 -> Out1/1
  In3/1 -> If/1, If Action Subsystem/1(In1), If Action Subsystem1/1(In1), If Action Subsystem2/1(In1), If Action Subsystem3/1(In1)
  If Action Subsystem2/1(Out1) -> Merge/3
  If Action Subsystem1/1(Out1) -> Merge/2
  If Action Subsystem3/1(Out1) -> Merge/4
  If Action Subsystem/1(Out1) -> Merge/1
  If/4 -> If Action Subsystem3/Action
  If/3 -> If Action Subsystem2/Action
  If/2 -> If Action Subsystem1/Action
  If/1 -> If Action Subsystem/Action

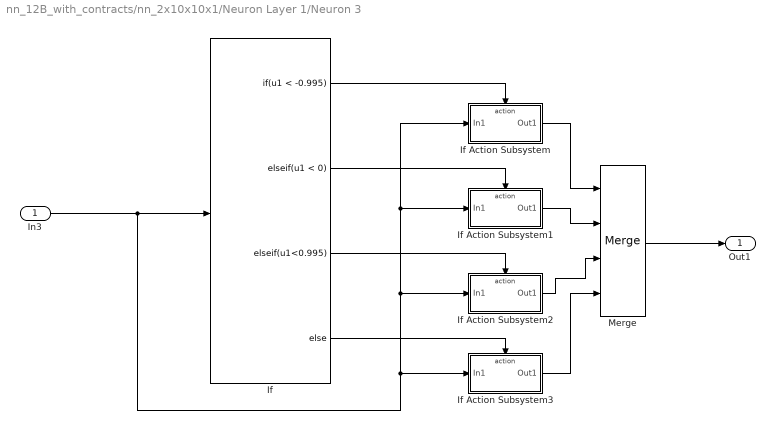
== system nn_12B_with_contracts/nn_2x10x10x1/Neuron Layer 1/Neuron 3 ==
  In3 : Inport
  If : If  IfExpression=u1 < -0.995  ElseIfExpressions=u1 < 0, u1<0.995
  If Action Subsystem : Subsystem  TreatAsAtomicUnit=on
  If Action Subsystem1 : Subsystem  TreatAsAtomicUnit=on
  If Action Subsystem2 : Subsystem  TreatAsAtomicUnit=on
  If Action Subsystem3 : Subsystem  TreatAsAtomicUnit=on
  Merge : Merge  Inputs=4
  Out1 : Outport  VectorParamsAs1DForOutWhenUnconnected=off
  wires:
  If/1 -> If Action Subsystem/Action
  If/2 -> If Action Subsystem1/Action
  If/3 -> If Action Subsystem2/Action
  If/4 -> If Action Subsystem3/Action
  If Action Subsystem/1(Out1) -> Merge/1
  If Action Subsystem3/1(Out1) -> Merge/4
  If Action Subsystem1/1(Out1) -> Merge/2
  If Action Subsystem2/1(Out1) -> Merge/3
  In3/1 -> If Action Subsystem3/1(In1), If Action Subsystem2/1(In1), If Action Subsystem1/1(In1), If Action Subsystem/1(In1), If/1
  Merge/1 -> Out1/1

== system nn_12B_with_contracts/nn_2x10x10x1/Neuron Layer 1/Neuron 4 ==
  In3 : Inport
  If : If  IfExpression=u1 < -0.995  ElseIfExpressions=u1 < 0, u1<0.995
  If Action Subsystem : Subsystem  TreatAsAtomicUnit=on
  If Action Subsystem1 : Subsystem  TreatAsAtomicUnit=on
  If Action Subsystem2 : Subsystem  TreatAsAtomicUnit=on
  If Action Subsystem3 : Subsystem  TreatAsAtomicUnit=on
  Merge : Merge  Inputs=4
  Out1 : Outport  VectorParamsAs1DForOutWhenUnconnected=off
  wires:
  If/1 -> If Action Subsystem/Action
  If/2 -> If Action Subsystem1/Action
  If/3 -> If Action Subsystem2/Action
  If/4 -> If Action Subsystem3/Action
  If Action Subsystem/1(Out1) -> Merge/1
  If Action Subsystem3/1(Out1) -> Merge/4
  If Action Subsystem1/1(Out1) -> Merge/2
  If Action Subsystem2/1(Out1) -> Merge/3
  In3/1 -> If Action Subsystem3/1(In1), If Action Subsystem2/1(In1), If Action Subsystem1/1(In1), If Action Subsystem/1(In1), If/1
  Merge/1 -> Out1/1

== system nn_12B_with_contracts/nn_2x10x10x1/Neuron Layer 1/Neuron 5 ==
  In3 : Inport
  If : If  IfExpression=u1 < -0.995  ElseIfExpressions=u1 < 0, u1<0.995
  If Action Subsystem : Subsystem  TreatAsAtomicUnit=on
  If Action Subsystem1 : Subsystem  TreatAsAtomicUnit=on
  If Action Subsystem2 : Subsystem  TreatAsAtomicUnit=on
  If Action Subsystem3 : Subsystem  TreatAsAtomicUnit=on
  Merge : Merge  Inputs=4
  Out1 : Outport  VectorParamsAs1DForOutWhenUnconnected=off
  wires:
  If/1 -> If Action Subsystem/Action
  If/2 -> If Action Subsystem1/Action
  If/3 -> If Action Subsystem2/Action
  If/4 -> If Action Subsystem3/Action
  If Action Subsystem/1(Out1) -> Merge/1
  If Action Subsystem3/1(Out1) -> Merge/4
  If Action Subsystem1/1(Out1) -> Merge/2
  If Action Subsystem2/1(Out1) -> Merge/3
  In3/1 -> If Action Subsystem3/1(In1), If Action Subsystem2/1(In1), If Action Subsystem1/1(In1), If Action Subsystem/1(In1), If/1
  Merge/1 -> Out1/1

== system nn_12B_with_contracts/nn_2x10x10x1/Neuron Layer 1/Neuron 6 ==
  In3 : Inport
  If : If  IfExpression=u1 < -0.995  ElseIfExpressions=u1 < 0, u1<0.995
  If Action Subsystem : Subsystem  TreatAsAtomicUnit=on
  If Action Subsystem1 : Subsystem  TreatAsAtomicUnit=on
  If Action Subsystem2 : Subsystem  TreatAsAtomicUnit=on
  If Action Subsystem3 : Subsystem  TreatAsAtomicUnit=on
  Merge : Merge  Inputs=4
  Out1 : Outport  VectorParamsAs1DForOutWhenUnconnected=off
  wires:
  Merge/1 -> Out1/1
  In3/1 -> If/1, If Action Subsystem/1(In1), If Action Subsystem1/1(In1), If Action Subsystem2/1(In1), If Action Subsystem3/1(In1)
  If Action Subsystem2/1(Out1) -> Merge/3
  If Action Subsystem1/1(Out1) -> Merge/2
  If Action Subsystem3/1(Out1) -> Merge/4
  If Action Subsystem/1(Out1) -> Merge/1
  If/4 -> If Action Subsystem3/Action
  If/3 -> If Action Subsystem2/Action
  If/2 -> If Action Subsystem1/Action
  If/1 -> If Action Subsystem/Action

== system nn_12B_with_contracts/nn_2x10x10x1/Neuron Layer 1/Neuron 7 ==
  In3 : Inport
  If : If  IfExpression=u1 < -0.995  ElseIfExpressions=u1 < 0, u1<0.995
  If Action Subsystem : Subsystem  TreatAsAtomicUnit=on
  If Action Subsystem1 : Subsystem  TreatAsAtomicUnit=on
  If Action Subsystem2 : Subsystem  TreatAsAtomicUnit=on
  If Action Subsystem3 : Subsystem  TreatAsAtomicUnit=on
  Merge : Merge  Inputs=4
  Out1 : Outport  VectorParamsAs1DForOutWhenUnconnected=off
  wires:
  If/1 -> If Action Subsystem/Action
  If/2 -> If Action Subsystem1/Action
  If/3 -> If Action Subsystem2/Action
  If/4 -> If Action Subsystem3/Action
  If Action Subsystem/1(Out1) -> Merge/1
  If Action Subsystem3/1(Out1) -> Merge/4
  If Action Subsystem1/1(Out1) -> Merge/2
  If Action Subsystem2/1(Out1) -> Merge/3
  In3/1 -> If Action Subsystem3/1(In1), If Action Subsystem2/1(In1), If Action Subsystem1/1(In1), If Action Subsystem/1(In1), If/1
  Merge/1 -> Out1/1

== system nn_12B_with_contracts/nn_2x10x10x1/Neuron Layer 1/Neuron 8 ==
  In3 : Inport
  If : If  IfExpression=u1 < -0.995  ElseIfExpressions=u1 < 0, u1<0.995
  If Action Subsystem : Subsystem  TreatAsAtomicUnit=on
  If Action Subsystem1 : Subsystem  TreatAsAtomicUnit=on
  If Action Subsystem2 : Subsystem  TreatAsAtomicUnit=on
  If Action Subsystem3 : Subsystem  TreatAsAtomicUnit=on
  Merge : Merge  Inputs=4
  Out1 : Outport  VectorParamsAs1DForOutWhenUnconnected=off
  wires:
  If/1 -> If Action Subsystem/Action
  If/2 -> If Action Subsystem1/Action
  If/3 -> If Action Subsystem2/Action
  If/4 -> If Action Subsystem3/Action
  If Action Subsystem/1(Out1) -> Merge/1
  If Action Subsystem3/1(Out1) -> Merge/4
  If Action Subsystem1/1(Out1) -> Merge/2
  If Action Subsystem2/1(Out1) -> Merge/3
  In3/1 -> If Action Subsystem3/1(In1), If Action Subsystem2/1(In1), If Action Subsystem1/1(In1), If Action Subsystem/1(In1), If/1
  Merge/1 -> Out1/1

== system nn_12B_with_contracts/nn_2x10x10x1/Neuron Layer 1/Neuron 9 ==
  In3 : Inport
  If : If  IfExpression=u1 < -0.995  ElseIfExpressions=u1 < 0, u1<0.995
  If Action Subsystem : Subsystem  TreatAsAtomicUnit=on
  If Action Subsystem1 : Subsystem  TreatAsAtomicUnit=on
  If Action Subsystem2 : Subsystem  TreatAsAtomicUnit=on
  If Action Subsystem3 : Subsystem  TreatAsAtomicUnit=on
  Merge : Merge  Inputs=4
  Out1 : Outport  VectorParamsAs1DForOutWhenUnconnected=off
  wires:
  If/1 -> If Action Subsystem/Action
  If/2 -> If Action Subsystem1/Action
  If/3 -> If Action Subsystem2/Action
  If/4 -> If Action Subsystem3/Action
  If Action Subsystem/1(Out1) -> Merge/1
  If Action Subsystem3/1(Out1) -> Merge/4
  If Action Subsystem1/1(Out1) -> Merge/2
  If Action Subsystem2/1(Out1) -> Merge/3
  In3/1 -> If Action Subsystem3/1(In1), If Action Subsystem2/1(In1), If Action Subsystem1/1(In1), If Action Subsystem/1(In1), If/1
  Merge/1 -> Out1/1

== system nn_12B_with_contracts/nn_2x10x10x1/Neuron Layer 2/Neuron 1 ==
  In3 : Inport
  If : If  IfExpression=u1 < -0.995  ElseIfExpressions=u1 < 0, u1<0.995
  If Action Subsystem : Subsystem  TreatAsAtomicUnit=on
  If Action Subsystem1 : Subsystem  TreatAsAtomicUnit=on
  If Action Subsystem2 : Subsystem  TreatAsAtomicUnit=on
  If Action Subsystem3 : Subsystem  TreatAsAtomicUnit=on
  Merge : Merge  Inputs=4
  Out1 : Outport  VectorParamsAs1DForOutWhenUnconnected=off
  wires:
  If/1 -> If Action Subsystem/Action
  If/2 -> If Action Subsystem1/Action
  If/3 -> If Action Subsystem2/Action
  If/4 -> If Action Subsystem3/Action
  If Action Subsystem/1(Out1) -> Merge/1
  If Action Subsystem3/1(Out1) -> Merge/4
  If Action Subsystem1/1(Out1) -> Merge/2
  If Action Subsystem2/1(Out1) -> Merge/3
  In3/1 -> If Action Subsystem3/1(In1), If Action Subsystem2/1(In1), If Action Subsystem1/1(In1), If Action Subsystem/1(In1), If/1
  Merge/1 -> Out1/1

== system nn_12B_with_contracts/nn_2x10x10x1/Neuron Layer 2/Neuron 10 ==
  In3 : Inport
  If : If  IfExpression=u1 < -0.995  ElseIfExpressions=u1 < 0, u1<0.995
  If Action Subsystem : Subsystem  TreatAsAtomicUnit=on
  If Action Subsystem1 : Subsystem  TreatAsAtomicUnit=on
  If Action Subsystem2 : Subsystem  TreatAsAtomicUnit=on
  If Action Subsystem3 : Subsystem  TreatAsAtomicUnit=on
  Merge : Merge  Inputs=4
  Out1 : Outport  VectorParamsAs1DForOutWhenUnconnected=off
  wires:
  Merge/1 -> Out1/1
  In3/1 -> If/1, If Action Subsystem/1(In1), If Action Subsystem1/1(In1), If Action Subsystem2/1(In1), If Action Subsystem3/1(In1)
  If Action Subsystem2/1(Out1) -> Merge/3
  If Action Subsystem1/1(Out1) -> Merge/2
  If Action Subsystem3/1(Out1) -> Merge/4
  If Action Subsystem/1(Out1) -> Merge/1
  If/4 -> If Action Subsystem3/Action
  If/3 -> If Action Subsystem2/Action
  If/2 -> If Action Subsystem1/Action
  If/1 -> If Action Subsystem/Action

== system nn_12B_with_contracts/nn_2x10x10x1/Neuron Layer 2/Neuron 2 ==
  In3 : Inport
  If : If  IfExpression=u1 < -0.995  ElseIfExpressions=u1 < 0, u1<0.995
  If Action Subsystem : Subsystem  TreatAsAtomicUnit=on
  If Action Subsystem1 : Subsystem  TreatAsAtomicUnit=on
  If Action Subsystem2 : Subsystem  TreatAsAtomicUnit=on
  If Action Subsystem3 : Subsystem  TreatAsAtomicUnit=on
  Merge : Merge  Inputs=4
  Out1 : Outport  VectorParamsAs1DForOutWhenUnconnected=off
  wires:
  Merge/1 -> Out1/1
  In3/1 -> If/1, If Action Subsystem/1(In1), If Action Subsystem1/1(In1), If Action Subsystem2/1(In1), If Action Subsystem3/1(In1)
  If Action Subsystem2/1(Out1) -> Merge/3
  If Action Subsystem1/1(Out1) -> Merge/2
  If Action Subsystem3/1(Out1) -> Merge/4
  If Action Subsystem/1(Out1) -> Merge/1
  If/4 -> If Action Subsystem3/Action
  If/3 -> If Action Subsystem2/Action
  If/2 -> If Action Subsystem1/Action
  If/1 -> If Action Subsystem/Action

== system nn_12B_with_contracts/nn_2x10x10x1/Neuron Layer 2/Neuron 3 ==
  In3 : Inport
  If : If  IfExpression=u1 < -0.995  ElseIfExpressions=u1 < 0, u1<0.995
  If Action Subsystem : Subsystem  TreatAsAtomicUnit=on
  If Action Subsystem1 : Subsystem  TreatAsAtomicUnit=on
  If Action Subsystem2 : Subsystem  TreatAsAtomicUnit=on
  If Action Subsystem3 : Subsystem  TreatAsAtomicUnit=on
  Merge : Merge  Inputs=4
  Out1 : Outport  VectorParamsAs1DForOutWhenUnconnected=off
  wires:
  If/1 -> If Action Subsystem/Action
  If/2 -> If Action Subsystem1/Action
  If/3 -> If Action Subsystem2/Action
  If/4 -> If Action Subsystem3/Action
  If Action Subsystem/1(Out1) -> Merge/1
  If Action Subsystem3/1(Out1) -> Merge/4
  If Action Subsystem1/1(Out1) -> Merge/2
  If Action Subsystem2/1(Out1) -> Merge/3
  In3/1 -> If Action Subsystem3/1(In1), If Action Subsystem2/1(In1), If Action Subsystem1/1(In1), If Action Subsystem/1(In1), If/1
  Merge/1 -> Out1/1

== system nn_12B_with_contracts/nn_2x10x10x1/Neuron Layer 2/Neuron 4 ==
  In3 : Inport
  If : If  IfExpression=u1 < -0.995  ElseIfExpressions=u1 < 0, u1<0.995
  If Action Subsystem : Subsystem  TreatAsAtomicUnit=on
  If Action Subsystem1 : Subsystem  TreatAsAtomicUnit=on
  If Action Subsystem2 : Subsystem  TreatAsAtomicUnit=on
  If Action Subsystem3 : Subsystem  TreatAsAtomicUnit=on
  Merge : Merge  Inputs=4
  Out1 : Outport  VectorParamsAs1DForOutWhenUnconnected=off
  wires:
  If/1 -> If Action Subsystem/Action
  If/2 -> If Action Subsystem1/Action
  If/3 -> If Action Subsystem2/Action
  If/4 -> If Action Subsystem3/Action
  If Action Subsystem/1(Out1) -> Merge/1
  If Action Subsystem3/1(Out1) -> Merge/4
  If Action Subsystem1/1(Out1) -> Merge/2
  If Action Subsystem2/1(Out1) -> Merge/3
  In3/1 -> If Action Subsystem3/1(In1), If Action Subsystem2/1(In1), If Action Subsystem1/1(In1), If Action Subsystem/1(In1), If/1
  Merge/1 -> Out1/1

== system nn_12B_with_contracts/nn_2x10x10x1/Neuron Layer 2/Neuron 5 ==
  In3 : Inport
  If : If  IfExpression=u1 < -0.995  ElseIfExpressions=u1 < 0, u1<0.995
  If Action Subsystem : Subsystem  TreatAsAtomicUnit=on
  If Action Subsystem1 : Subsystem  TreatAsAtomicUnit=on
  If Action Subsystem2 : Subsystem  TreatAsAtomicUnit=on
  If Action Subsystem3 : Subsystem  TreatAsAtomicUnit=on
  Merge : Merge  Inputs=4
  Out1 : Outport  VectorParamsAs1DForOutWhenUnconnected=off
  wires:
  If/1 -> If Action Subsystem/Action
  If/2 -> If Action Subsystem1/Action
  If/3 -> If Action Subsystem2/Action
  If/4 -> If Action Subsystem3/Action
  If Action Subsystem/1(Out1) -> Merge/1
  If Action Subsystem3/1(Out1) -> Merge/4
  If Action Subsystem1/1(Out1) -> Merge/2
  If Action Subsystem2/1(Out1) -> Merge/3
  In3/1 -> If Action Subsystem3/1(In1), If Action Subsystem2/1(In1), If Action Subsystem1/1(In1), If Action Subsystem/1(In1), If/1
  Merge/1 -> Out1/1

== system nn_12B_with_contracts/nn_2x10x10x1/Neuron Layer 2/Neuron 6 ==
  In3 : Inport
  If : If  IfExpression=u1 < -0.995  ElseIfExpressions=u1 < 0, u1<0.995
  If Action Subsystem : Subsystem  TreatAsAtomicUnit=on
  If Action Subsystem1 : Subsystem  TreatAsAtomicUnit=on
  If Action Subsystem2 : Subsystem  TreatAsAtomicUnit=on
  If Action Subsystem3 : Subsystem  TreatAsAtomicUnit=on
  Merge : Merge  Inputs=4
  Out1 : Outport  VectorParamsAs1DForOutWhenUnconnected=off
  wires:
  Merge/1 -> Out1/1
  In3/1 -> If/1, If Action Subsystem/1(In1), If Action Subsystem1/1(In1), If Action Subsystem2/1(In1), If Action Subsystem3/1(In1)
  If Action Subsystem2/1(Out1) -> Merge/3
  If Action Subsystem1/1(Out1) -> Merge/2
  If Action Subsystem3/1(Out1) -> Merge/4
  If Action Subsystem/1(Out1) -> Merge/1
  If/4 -> If Action Subsystem3/Action
  If/3 -> If Action Subsystem2/Action
  If/2 -> If Action Subsystem1/Action
  If/1 -> If Action Subsystem/Action

== system nn_12B_with_contracts/nn_2x10x10x1/Neuron Layer 2/Neuron 7 ==
  In3 : Inport
  If : If  IfExpression=u1 < -0.995  ElseIfExpressions=u1 < 0, u1<0.995
  If Action Subsystem : Subsystem  TreatAsAtomicUnit=on
  If Action Subsystem1 : Subsystem  TreatAsAtomicUnit=on
  If Action Subsystem2 : Subsystem  TreatAsAtomicUnit=on
  If Action Subsystem3 : Subsystem  TreatAsAtomicUnit=on
  Merge : Merge  Inputs=4
  Out1 : Outport  VectorParamsAs1DForOutWhenUnconnected=off
  wires:
  If/1 -> If Action Subsystem/Action
  If/2 -> If Action Subsystem1/Action
  If/3 -> If Action Subsystem2/Action
  If/4 -> If Action Subsystem3/Action
  If Action Subsystem/1(Out1) -> Merge/1
  If Action Subsystem3/1(Out1) -> Merge/4
  If Action Subsystem1/1(Out1) -> Merge/2
  If Action Subsystem2/1(Out1) -> Merge/3
  In3/1 -> If Action Subsystem3/1(In1), If Action Subsystem2/1(In1), If Action Subsystem1/1(In1), If Action Subsystem/1(In1), If/1
  Merge/1 -> Out1/1

== system nn_12B_with_contracts/nn_2x10x10x1/Neuron Layer 2/Neuron 8 ==
  In3 : Inport
  If : If  IfExpression=u1 < -0.995  ElseIfExpressions=u1 < 0, u1<0.995
  If Action Subsystem : Subsystem  TreatAsAtomicUnit=on
  If Action Subsystem1 : Subsystem  TreatAsAtomicUnit=on
  If Action Subsystem2 : Subsystem  TreatAsAtomicUnit=on
  If Action Subsystem3 : Subsystem  TreatAsAtomicUnit=on
  Merge : Merge  Inputs=4
  Out1 : Outport  VectorParamsAs1DForOutWhenUnconnected=off
  wires:
  If/1 -> If Action Subsystem/Action
  If/2 -> If Action Subsystem1/Action
  If/3 -> If Action Subsystem2/Action
  If/4 -> If Action Subsystem3/Action
  If Action Subsystem/1(Out1) -> Merge/1
  If Action Subsystem3/1(Out1) -> Merge/4
  If Action Subsystem1/1(Out1) -> Merge/2
  If Action Subsystem2/1(Out1) -> Merge/3
  In3/1 -> If Action Subsystem3/1(In1), If Action Subsystem2/1(In1), If Action Subsystem1/1(In1), If Action Subsystem/1(In1), If/1
  Merge/1 -> Out1/1

== system nn_12B_with_contracts/nn_2x10x10x1/Neuron Layer 2/Neuron 9 ==
  In3 : Inport
  If : If  IfExpression=u1 < -0.995  ElseIfExpressions=u1 < 0, u1<0.995
  If Action Subsystem : Subsystem  TreatAsAtomicUnit=on
  If Action Subsystem1 : Subsystem  TreatAsAtomicUnit=on
  If Action Subsystem2 : Subsystem  TreatAsAtomicUnit=on
  If Action Subsystem3 : Subsystem  TreatAsAtomicUnit=on
  Merge : Merge  Inputs=4
  Out1 : Outport  VectorParamsAs1DForOutWhenUnconnected=off
  wires:
  If/1 -> If Action Subsystem/Action
  If/2 -> If Action Subsystem1/Action
  If/3 -> If Action Subsystem2/Action
  If/4 -> If Action Subsystem3/Action
  If Action Subsystem/1(Out1) -> Merge/1
  If Action Subsystem3/1(Out1) -> Merge/4
  If Action Subsystem1/1(Out1) -> Merge/2
  If Action Subsystem2/1(Out1) -> Merge/3
  In3/1 -> If Action Subsystem3/1(In1), If Action Subsystem2/1(In1), If Action Subsystem1/1(In1), If Action Subsystem/1(In1), If/1
  Merge/1 -> Out1/1

== system nn_12B_with_contracts/nn_2x10x10x1/Neuron Layer 1/Neuron 1/If Action Subsystem ==
  In1 : Inport
  Action Port : ActionPort  ActionPortLabel=if { }
  Sum : Sum  Inputs=|+-
  bias1 : Constant  Value=0.990025
  weight1 : Gain  Gain=0.01
  Out1 : Outport  VectorParamsAs1DForOutWhenUnconnected=off
  wires:
  bias1/1 -> Sum/2
  weight1/1 -> Sum/1
  In1/1 -> weight1/1
  Sum/1 -> Out1/1

== system nn_12B_with_contracts/nn_2x10x10x1/Neuron Layer 1/Neuron 1/If Action Subsystem1 ==
  In1 : Inport
  Action Port : ActionPort  ActionPortLabel=elseif { }
  Product1 : Product  RndMeth=Zero
  Sum3 : Sum  Inputs=|++
  bias4 : Constant  Value=2
  Out1 : Outport  VectorParamsAs1DForOutWhenUnconnected=off
  wires:
  In1/1 -> Product1/1, Sum3/1
  bias4/1 -> Sum3/2
  Sum3/1 -> Product1/2
  Product1/1 -> Out1/1

== system nn_12B_with_contracts/nn_2x10x10x1/Neuron Layer 1/Neuron 1/If Action Subsystem2 ==
  In1 : Inport
  Action Port : ActionPort  ActionPortLabel=elseif { }
  Product1 : Product  RndMeth=Zero
  Sum3 : Sum  Inputs=|-+
  bias4 : Constant  Value=2
  Out1 : Outport  VectorParamsAs1DForOutWhenUnconnected=off
  wires:
  Product1/1 -> Out1/1
  Sum3/1 -> Product1/2
  bias4/1 -> Sum3/2
  In1/1 -> Sum3/1, Product1/1

== system nn_12B_with_contracts/nn_2x10x10x1/Neuron Layer 1/Neuron 1/If Action Subsystem3 ==
  In1 : Inport
  Action Port : ActionPort  ActionPortLabel=else { }
  Sum : Sum  Inputs=|++
  bias1 : Constant  Value=0.990025
  weight1 : Gain  Gain=0.01
  Out1 : Outport  VectorParamsAs1DForOutWhenUnconnected=off
  wires:
  bias1/1 -> Sum/2
  weight1/1 -> Sum/1
  In1/1 -> weight1/1
  Sum/1 -> Out1/1

== system nn_12B_with_contracts/nn_2x10x10x1/Neuron Layer 1/Neuron 10/If Action Subsystem ==
  In1 : Inport
  Action Port : ActionPort  ActionPortLabel=if { }
  Sum : Sum  Inputs=|+-
  bias1 : Constant  Value=0.990025
  weight1 : Gain  Gain=0.01
  Out1 : Outport  VectorParamsAs1DForOutWhenUnconnected=off
  wires:
  Sum/1 -> Out1/1
  In1/1 -> weight1/1
  weight1/1 -> Sum/1
  bias1/1 -> Sum/2

== system nn_12B_with_contracts/nn_2x10x10x1/Neuron Layer 1/Neuron 10/If Action Subsystem1 ==
  In1 : Inport
  Action Port : ActionPort  ActionPortLabel=elseif { }
  Product1 : Product  RndMeth=Zero
  Sum3 : Sum  Inputs=|++
  bias4 : Constant  Value=2
  Out1 : Outport  VectorParamsAs1DForOutWhenUnconnected=off
  wires:
  Product1/1 -> Out1/1
  Sum3/1 -> Product1/2
  bias4/1 -> Sum3/2
  In1/1 -> Sum3/1, Product1/1

== system nn_12B_with_contracts/nn_2x10x10x1/Neuron Layer 1/Neuron 10/If Action Subsystem2 ==
  In1 : Inport
  Action Port : ActionPort  ActionPortLabel=elseif { }
  Product1 : Product  RndMeth=Zero
  Sum3 : Sum  Inputs=|-+
  bias4 : Constant  Value=2
  Out1 : Outport  VectorParamsAs1DForOutWhenUnconnected=off
  wires:
  In1/1 -> Product1/1, Sum3/1
  bias4/1 -> Sum3/2
  Sum3/1 -> Product1/2
  Product1/1 -> Out1/1

== system nn_12B_with_contracts/nn_2x10x10x1/Neuron Layer 1/Neuron 10/If Action Subsystem3 ==
  In1 : Inport
  Action Port : ActionPort  ActionPortLabel=else { }
  Sum : Sum  Inputs=|++
  bias1 : Constant  Value=0.990025
  weight1 : Gain  Gain=0.01
  Out1 : Outport  VectorParamsAs1DForOutWhenUnconnected=off
  wires:
  Sum/1 -> Out1/1
  In1/1 -> weight1/1
  weight1/1 -> Sum/1
  bias1/1 -> Sum/2

== system nn_12B_with_contracts/nn_2x10x10x1/Neuron Layer 1/Neuron 2/If Action Subsystem ==
  In1 : Inport
  Action Port : ActionPort  ActionPortLabel=if { }
  Sum : Sum  Inputs=|+-
  bias1 : Constant  Value=0.990025
  weight1 : Gain  Gain=0.01
  Out1 : Outport  VectorParamsAs1DForOutWhenUnconnected=off
  wires:
  Sum/1 -> Out1/1
  In1/1 -> weight1/1
  weight1/1 -> Sum/1
  bias1/1 -> Sum/2
